simulink model "Working_model_LastVersion24_June_"  (R2020a)
settings: Solver=VariableStepAuto  StartTime=0.0  StopTime=20  RelTol=1e-3
values from neighbouring files (symbols this model uses):
  g = 9.81    [Working_model_LastVersion24_June.m]    (also in model_and_controller.m)
  K = (m_b/(m_b+(Ib/r_b^2)))    (= 0.714285714286)    [Working_model_LastVersion24_June.m]    (also in model_and_controller.m)
  Ts_Outer = 0.1    [Working_model_LastVersion24_June.m]    (also in model_and_controller.m)
undefined symbols (not defined in the file or in its folder): denc_mi, denco12_dis_des, denF, denp_mi, numc_mi, numco12_dis_des, numF, nump_mi
libraries: simulink x1
settings Model: PacingRate=0.500000  Creator=elakz  LastModifiedBy=elakz

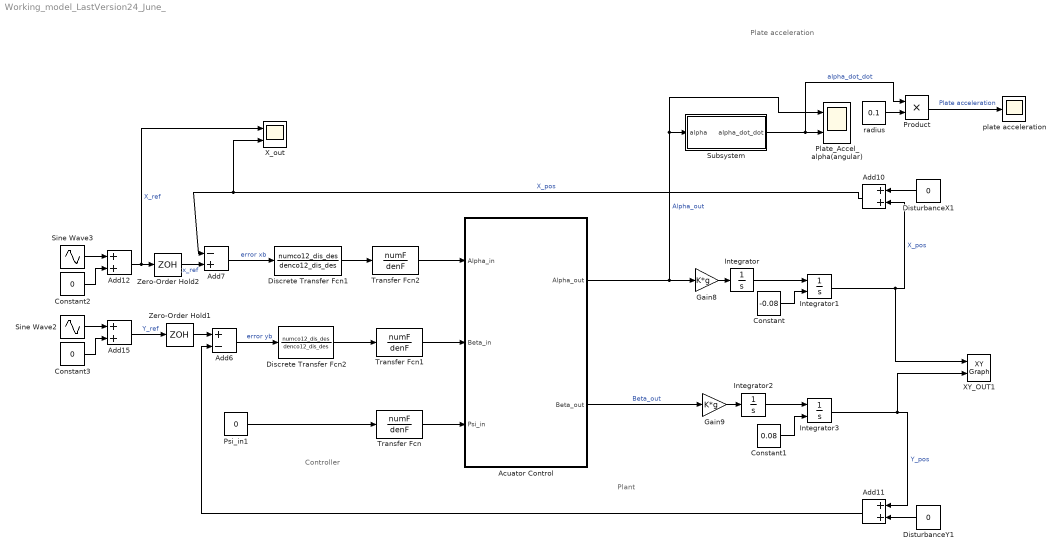
== system Working_model_LastVersion24_June_ ==
  note: Controller
  note: Plant
  note: Plate acceleration
  Acuator Control : Subsystem
  Add{10..12,15} (4 alike) : Sum
  Add6 : Sum  Inputs=+-
  Add7 : Sum  Inputs=-+
  Constant : Constant  Value=-0.08
  Constant1 : Constant  Value=0.08
  Constant2 : Constant  Value=0
  Constant3 : Constant  Value=0
  Discrete Transfer Fcn1 : DiscreteTransferFcn  Numerator=numco12_dis_des  Denominator=denco12_dis_des
  Discrete Transfer Fcn2 : DiscreteTransferFcn  Numerator=numco12_dis_des  Denominator=denco12_dis_des
  DisturbanceX1 : Constant  Value=0
  DisturbanceY1 : Constant  Value=0
  Gain8 : Gain  Gain=K*g
  Gain9 : Gain  Gain=K*g
  Integrator : Integrator
  Integrator1 : Integrator  InitialConditionSource=external  InitialCondition=0.01
  Integrator2 : Integrator
  Integrator3 : Integrator  InitialConditionSource=external  InitialCondition=0.01
  Plate_Accel_alpha(angular) : Scope  NumInputPorts=2
  Product : Product
  Psi_in1 : Constant  Value=0
  Sine Wave2 : Sin  Amplitude=0.1  Frequency=2*pi*0.6  Phase=pi/2  SampleTime=0
  Sine Wave3 : Sin  Amplitude=0.1  Frequency=2*pi*0.6  SampleTime=0
  Subsystem : Subsystem
  Transfer Fcn : TransferFcn  Numerator=numF  Denominator=denF
  Transfer Fcn1 : TransferFcn  Numerator=numF  Denominator=denF
  Transfer Fcn2 : TransferFcn  Numerator=numF  Denominator=denF
  XY_OUT1 : simulink/Sinks/XY Graph  xmin=-0.2  xmax=0.2  ymin=-0.2  ymax=0.2  st=-1
  X_out : Scope  NumInputPorts=2
  Zero-Order Hold1 : ZeroOrderHold  SampleTime=Ts_Outer
  Zero-Order Hold2 : ZeroOrderHold  SampleTime=Ts_Outer
  plate acceleration : Scope
  radius : Constant  Value=0.1
  wires:
  Constant3/1 -> Add15/2
  Constant/1 -> Integrator1/2
  Zero-Order Hold1/1 -> Add6/1
  Integrator3/1 -> XY_OUT1/2, Add11/1  "Y_pos"
  DisturbanceX1/1 -> Add10/1
  Add11/1 -> Add6/2
  Gain8/1 -> Integrator/1
  Add7/1 -> Discrete Transfer Fcn1/1  "error xb"
  Add6/1 -> Discrete Transfer Fcn2/1  "error yb"
  DisturbanceY1/1 -> Add11/2
  Gain9/1 -> Integrator2/1
  Zero-Order Hold2/1 -> Add7/2  "x_ref"
  Integrator1/1 -> XY_OUT1/1, Add10/2  "X_pos"
  Integrator/1 -> Integrator1/1
  Subsystem/1(alpha_dot_dot) -> Product/1, Plate_Accel_alpha(angular)/2  "alpha_dot_dot"
  Constant2/1 -> Add12/2
  Constant1/1 -> Integrator3/2
  Sine Wave3/1 -> Add12/1
  Integrator2/1 -> Integrator3/1
  Add10/1 -> X_out/2, Add7/1  "X_pos"
  Sine Wave2/1 -> Add15/1
  Acuator Control/1(Alpha_out) -> Subsystem/1(alpha), Plate_Accel_alpha(angular)/1, Gain8/1  "Alpha_out"
  Acuator Control/2(Beta_out) -> Gain9/1  "Beta_out"
  Add12/1 -> X_out/1, Zero-Order Hold2/1  "X_ref"
  Transfer Fcn2/1 -> Acuator Control/1(Alpha_in)
  Discrete Transfer Fcn1/1 -> Transfer Fcn2/1
  Transfer Fcn1/1 -> Acuator Control/2(Beta_in)
  Discrete Transfer Fcn2/1 -> Transfer Fcn1/1
  Psi_in1/1 -> Transfer Fcn/1
  Transfer Fcn/1 -> Acuator Control/3(Psi_in)
  radius/1 -> Product/2
  Product/1 -> plate acceleration/1  "Plate acceleration"
  Add15/1 -> Zero-Order Hold1/1  "Y_ref"

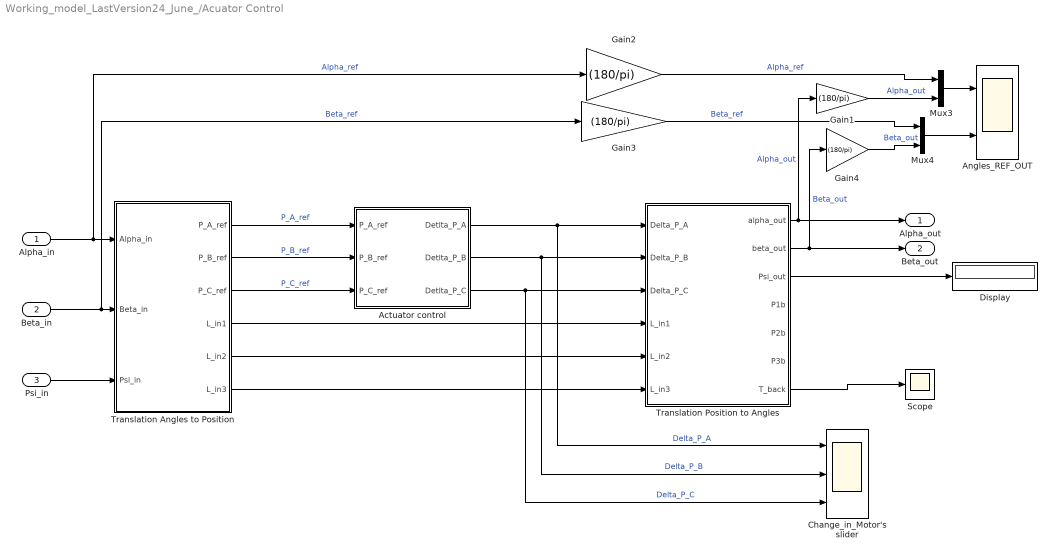
== system Working_model_LastVersion24_June_/Acuator Control ==
  Alpha_in : Inport
  Beta_in : Inport  Port=2
  Psi_in : Inport  Port=3
  Actuator control : Subsystem
  Angles_REF_OUT : Scope  NumInputPorts=2
  Change_in_Motor's slider : Scope  NumInputPorts=3
  Display : Display
  Gain{1..4} (4 alike) : Gain  Gain=(180/pi)
  Mux3 : Mux  Inputs=2
  Mux4 : Mux  Inputs=2
  Scope : Scope
  Translation Angles to Position : Subsystem
  Translation Position to Angles : Subsystem
  Alpha_out : Outport  VectorParamsAs1DForOutWhenUnconnected=off
  Beta_out : Outport  Port=2  VectorParamsAs1DForOutWhenUnconnected=off
  wires:
  Translation Angles to Position/6(L_in3) -> Translation Position to Angles/6(L_in3)
  Translation Angles to Position/1(P_A_ref) -> Actuator control/1(P_A_ref)  "P_A_ref"
  Actuator control/2(Detlta_P_B) -> Change_in_Motor's slider/2, Translation Position to Angles/2(Delta_P_B)  "Delta_P_B"
  Actuator control/3(Detlta_P_C) -> Change_in_Motor's slider/3, Translation Position to Angles/3(Delta_P_C)  "Delta_P_C"
  Translation Angles to Position/2(P_B_ref) -> Actuator control/2(P_B_ref)  "P_B_ref"
  Translation Angles to Position/5(L_in2) -> Translation Position to Angles/5(L_in2)
  Translation Angles to Position/3(P_C_ref) -> Actuator control/3(P_C_ref)  "P_C_ref"
  Translation Angles to Position/4(L_in1) -> Translation Position to Angles/4(L_in1)
  Actuator control/1(Detlta_P_A) -> Change_in_Motor's slider/1, Translation Position to Angles/1(Delta_P_A)  "Delta_P_A"
  Beta_in/1 -> Gain3/1, Translation Angles to Position/2(Beta_in)  "Beta_ref"
  Psi_in/1 -> Translation Angles to Position/3(Psi_in)
  Translation Position to Angles/2(beta_out) -> Gain4/1, Beta_out/1  "Beta_out"
  Translation Position to Angles/1(alpha_out) -> Gain1/1, Alpha_out/1  "Alpha_out"
  Alpha_in/1 -> Gain2/1, Translation Angles to Position/1(Alpha_in)  "Alpha_ref"
  Translation Position to Angles/3(Psi_out) -> Display/1
  Mux3/1 -> Angles_REF_OUT/1
  Mux4/1 -> Angles_REF_OUT/2
  Gain2/1 -> Mux3/1  "Alpha_ref"
  Gain1/1 -> Mux3/2  "Alpha_out"
  Gain3/1 -> Mux4/1  "Beta_ref"
  Gain4/1 -> Mux4/2  "Beta_out"
  Translation Position to Angles/7(T_back) -> Scope/1

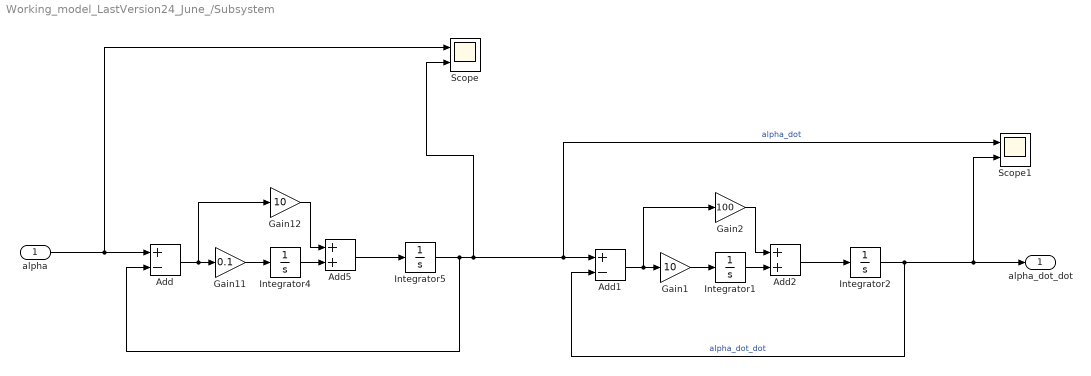
== system Working_model_LastVersion24_June_/Subsystem ==
  alpha : Inport
  Add : Sum  Inputs=+-
  Add1 : Sum  Inputs=+-
  Add2 : Sum
  Add5 : Sum
  Gain1 : Gain  Gain=10
  Gain11 : Gain  Gain=0.1
  Gain12 : Gain  Gain=10
  Gain2 : Gain  Gain=100
  Integrator{1..2,4..5} (4 alike) : Integrator
  Scope : Scope  NumInputPorts=2
  Scope1 : Scope  NumInputPorts=2
  alpha_dot_dot : Outport
  wires:
  Gain11/1 -> Integrator4/1
  Add5/1 -> Integrator5/1
  Gain1/1 -> Integrator1/1
  Integrator4/1 -> Add5/2
  Add/1 -> Gain12/1, Gain11/1
  Gain12/1 -> Add5/1
  Integrator2/1 -> alpha_dot_dot/1, Scope1/2, Add1/2  "alpha_dot_dot"
  Integrator5/1 -> Add/2, Scope/2, Scope1/1, Add1/1  "alpha_dot"
  Integrator1/1 -> Add2/2
  Add1/1 -> Gain2/1, Gain1/1
  Add2/1 -> Integrator2/1
  Gain2/1 -> Add2/1
  alpha/1 -> Scope/1, Add/1

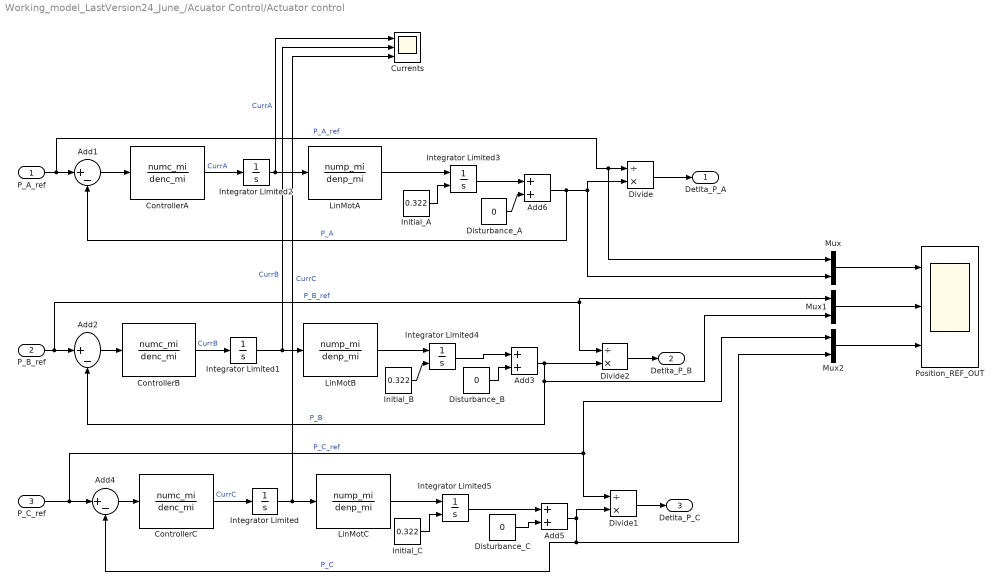
== system Working_model_LastVersion24_June_/Acuator Control/Actuator control ==
  P_A_ref : Inport
  P_B_ref : Inport  Port=2
  P_C_ref : Inport  Port=3
  Add1 : Sum  Inputs=|+-
  Add2 : Sum  Inputs=|+-
  Add3 : Sum
  Add4 : Sum  Inputs=|+-
  Add5 : Sum
  Add6 : Sum
  ControllerA : TransferFcn  Numerator=numc_mi  Denominator=denc_mi
  ControllerB : TransferFcn  Numerator=numc_mi  Denominator=denc_mi
  ControllerC : TransferFcn  Numerator=numc_mi  Denominator=denc_mi
  Currents : Scope  NumInputPorts=3
  Disturbance_A : Constant  Value=0
  Disturbance_B : Constant  Value=0
  Disturbance_C : Constant  Value=0
  Divide : Product  Inputs=/*
  Divide1 : Product  Inputs=/*
  Divide2 : Product  Inputs=/*
  Initial_A : Constant  Value=0.322
  Initial_B : Constant  Value=0.322
  Initial_C : Constant  Value=0.322
  Integrator Limited : Integrator  UpperSaturationLimit=3  LowerSaturationLimit=-3
  Integrator Limited1 : Integrator  UpperSaturationLimit=3  LowerSaturationLimit=-3
  Integrator Limited2 : Integrator  UpperSaturationLimit=3  LowerSaturationLimit=-3
  Integrator Limited3 : Integrator  InitialConditionSource=external  UpperSaturationLimit=1  LowerSaturationLimit=0
  Integrator Limited4 : Integrator  InitialConditionSource=external  UpperSaturationLimit=1  LowerSaturationLimit=0
  Integrator Limited5 : Integrator  InitialConditionSource=external  UpperSaturationLimit=1  LowerSaturationLimit=0
  LinMotA : TransferFcn  Numerator=nump_mi  Denominator=denp_mi
  LinMotB : TransferFcn  Numerator=nump_mi  Denominator=denp_mi
  LinMotC : TransferFcn  Numerator=nump_mi  Denominator=denp_mi
  Mux : Mux  Inputs=2
  Mux1 : Mux  Inputs=2
  Mux2 : Mux  Inputs=2
  Position_REF_OUT : Scope  NumInputPorts=3
  Detlta_P_A : Outport  VectorParamsAs1DForOutWhenUnconnected=off
  Detlta_P_B : Outport  Port=2  VectorParamsAs1DForOutWhenUnconnected=off
  Detlta_P_C : Outport  Port=3  VectorParamsAs1DForOutWhenUnconnected=off
  wires:
  Add6/1 -> Divide/2, Mux/2, Add1/2  "P_A"
  Disturbance_A/1 -> Add6/2
  Add1/1 -> ControllerA/1
  Add2/1 -> ControllerB/1
  Disturbance_B/1 -> Add3/2
  Add3/1 -> Add2/2, Mux1/2, Divide2/2  "P_B"
  Add4/1 -> ControllerC/1
  Disturbance_C/1 -> Add5/2
  Add5/1 -> Divide1/2, Add4/2, Mux2/2  "P_C"
  P_B_ref/1 -> Add2/1, Divide2/1, Mux1/1  "P_B_ref"
  P_A_ref/1 -> Add1/1, Mux/1, Divide/1  "P_A_ref"
  P_C_ref/1 -> Add4/1, Divide1/1, Mux2/1  "P_C_ref"
  Integrator Limited/1 -> Currents/3, LinMotC/1  "CurrC"
  ControllerC/1 -> Integrator Limited/1  "CurrC"
  Integrator Limited1/1 -> LinMotB/1, Currents/2  "CurrB"
  ControllerB/1 -> Integrator Limited1/1  "CurrB"
  Integrator Limited2/1 -> LinMotA/1, Currents/1  "CurrA"
  ControllerA/1 -> Integrator Limited2/1  "CurrA"
  Divide2/1 -> Detlta_P_B/1
  Divide1/1 -> Detlta_P_C/1
  Divide/1 -> Detlta_P_A/1
  Mux1/1 -> Position_REF_OUT/2
  Mux/1 -> Position_REF_OUT/1
  Mux2/1 -> Position_REF_OUT/3
  LinMotA/1 -> Integrator Limited3/1
  Integrator Limited3/1 -> Add6/1
  Initial_A/1 -> Integrator Limited3/2
  Initial_B/1 -> Integrator Limited4/2
  LinMotB/1 -> Integrator Limited4/1
  Integrator Limited4/1 -> Add3/1
  LinMotC/1 -> Integrator Limited5/1
  Initial_C/1 -> Integrator Limited5/2
  Integrator Limited5/1 -> Add5/1

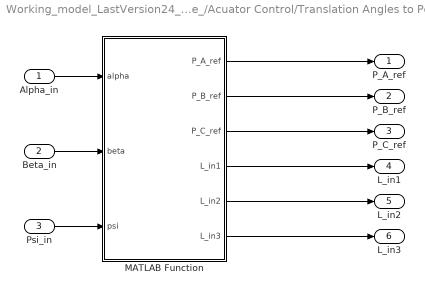
== system Working_model_LastVersion24_June_/Acuator Control/Translation Angles to Position ==
  Alpha_in : Inport
  Beta_in : Inport  Port=2
  Psi_in : Inport  Port=3
  MATLAB Function : MATLAB Function  TreatAsAtomicUnit=on
  P_A_ref : Outport  VectorParamsAs1DForOutWhenUnconnected=off
  P_B_ref : Outport  Port=2  VectorParamsAs1DForOutWhenUnconnected=off
  P_C_ref : Outport  Port=3  VectorParamsAs1DForOutWhenUnconnected=off
  L_in1 : Outport  Port=4  VectorParamsAs1DForOutWhenUnconnected=off
  L_in2 : Outport  Port=5  VectorParamsAs1DForOutWhenUnconnected=off
  L_in3 : Outport  Port=6  VectorParamsAs1DForOutWhenUnconnected=off
  wires:
  Alpha_in/1 -> MATLAB Function/1(alpha)
  MATLAB Function/6(L_in3) -> L_in3/1
  Psi_in/1 -> MATLAB Function/3(psi)
  MATLAB Function/5(L_in2) -> L_in2/1
  MATLAB Function/3(P_C_ref) -> P_C_ref/1
  MATLAB Function/2(P_B_ref) -> P_B_ref/1
  Beta_in/1 -> MATLAB Function/2(beta)
  MATLAB Function/4(L_in1) -> L_in1/1
  MATLAB Function/1(P_A_ref) -> P_A_ref/1

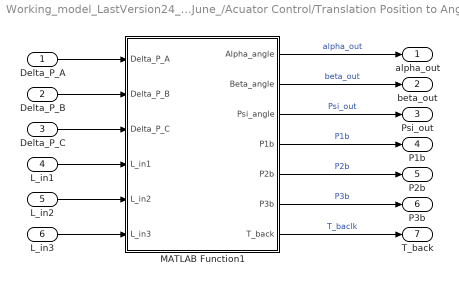
== system Working_model_LastVersion24_June_/Acuator Control/Translation Position to Angles ==
  Delta_P_A : Inport
  Delta_P_B : Inport  Port=2
  Delta_P_C : Inport  Port=3
  L_in1 : Inport  Port=4
  L_in2 : Inport  Port=5
  L_in3 : Inport  Port=6
  MATLAB Function1 : MATLAB Function  TreatAsAtomicUnit=on
  alpha_out : Outport  VectorParamsAs1DForOutWhenUnconnected=off
  beta_out : Outport  Port=2  VectorParamsAs1DForOutWhenUnconnected=off
  Psi_out : Outport  Port=3  VectorParamsAs1DForOutWhenUnconnected=off
  P1b : Outport  Port=4  VectorParamsAs1DForOutWhenUnconnected=off
  P2b : Outport  Port=5  VectorParamsAs1DForOutWhenUnconnected=off
  P3b : Outport  Port=6  VectorParamsAs1DForOutWhenUnconnected=off
  T_back : Outport  Port=7  VectorParamsAs1DForOutWhenUnconnected=off
  wires:
  MATLAB Function1/7(T_back) -> T_back/1  "T_baclk"
  MATLAB Function1/4(P1b) -> P1b/1  "P1b"
  MATLAB Function1/5(P2b) -> P2b/1  "P2b"
  Delta_P_C/1 -> MATLAB Function1/3(Delta_P_C)
  MATLAB Function1/6(P3b) -> P3b/1  "P3b"
  Delta_P_A/1 -> MATLAB Function1/1(Delta_P_A)
  Delta_P_B/1 -> MATLAB Function1/2(Delta_P_B)
  MATLAB Function1/3(Psi_angle) -> Psi_out/1  "Psi_out"
  MATLAB Function1/1(Alpha_angle) -> alpha_out/1  "alpha_out"
  MATLAB Function1/2(Beta_angle) -> beta_out/1  "beta_out"
  L_in3/1 -> MATLAB Function1/6(L_in3)
  L_in1/1 -> MATLAB Function1/4(L_in1)
  L_in2/1 -> MATLAB Function1/5(L_in2)

== matlab function Working_model_LastVersion24_June_/Acuator Control/Translation Angles to Position/MATLAB Function ==
  data: alpha input; beta input; psi input; P_A_ref output; P_B_ref output; P_C_ref output; L_in1 output; L_in2 output; L_in3 output
function [P_A_ref,P_B_ref,P_C_ref,L_in1,L_in2,L_in3] = myfunc(alpha,beta,psi)

%% Rotation matrices

%    Z rotation with angle  psi
RotZ  = [cos(psi) -sin(psi) 0;
         sin(psi)  cos(psi) 0;
          0          0      1]
      
%    Y rotation with angle beta+
RotY  = [cos(beta)       0         sin(beta);
             0           1             0    ;
         -sin(beta)      0        cos(beta)]
    
%    X rotation with angle alpha
RotX  = [1            0                 0    ;
         0        cos(alpha)      -sin(alpha);
         0        sin(alpha)       cos(alpha)]
Rot_BtoP = RotZ*RotY*RotX

%% Specification of the base plate and plate

%Location of motors on the base plate 
r_base = 0.17;               %radii of the base plate (m)
B1     = [r_base; 0; 0]      %position of motor wrt base plate origin
B2     = [-0.5*r_base; (sqrt(3)/2)*r_base; 0]  %120degrees wrt the position of first motor and base plate origin
B3     = [-0.5*r_base; -(sqrt(3)/2)*r_base; 0] %240 degrees wrt first motor and base plate origin

%Location of joints on the plate 
r_plate = 0.17;               %radii of the plate (m)
P1     = [r_plate; 0; 0]      %position of motor wrt base plate origin
P2     = [-0.5*r_plate; (sqrt(3)/2)*r_plate; 0]  %120degrees wrt the position of first motor and base plate origin
P3     = [-0.5*r_plate; -(sqrt(3)/2)*r_plate; 0] %240 degrees wrt first motor and base plate origin

% distance from base plate origin(OXYZ) to plate origin(oxyz)
T = [0; 0; 0.322]                     %30 cm height from (OXYZ) to (oxyz)

%% 
L_in1 = T + (Rot_BtoP*P1)-B1       %change of position of lin motor 1
P_A_ref = sqrt(L_in1(1,1)^2+L_in1(2,1)^2+L_in1(3,1)^2)   %length of L_in1 for passing to motor tf

L_in2 = T + (Rot_BtoP*P2)-B2
P_B_ref = sqrt(L_in2(1,1)^2+L_in2(2,1)^2+L_in2(3,1)^2)

L_in3 = T + (Rot_BtoP*P3)-B3 
P_C_ref = sqrt(L_in3(1,1)^2+L_in3(2,1)^2+L_in3(3,1)^2)
end

== matlab function Working_model_LastVersion24_June_/Acuator Control/Translation Position to Angles/MATLAB Function1 ==
  data: Delta_P_A input; Alpha_angle output; Delta_P_B input; Delta_P_C input; L_in1 input; L_in2 input; L_in3 input; Beta_angle output; Psi_angle output; P1b output; P2b output; P3b output; T_back output
function [Alpha_angle,Beta_angle,Psi_angle,P1b,P2b,P3b,T_back]      = myfunc(Delta_P_A,Delta_P_B,Delta_P_C,L_in1,L_in2,L_in3)



%% Specification of the base plate and plate

%Location of motors on the base plate 
r_base = 0.17;               %radii of the base plate (m)
B1     = [r_base; 0; 0]      %position of motor wrt base plate origin
B2     = [-0.5*r_base; (sqrt(3)/2)*r_base; 0]  %120degrees wrt the position of first motor and base plate origin
B3     = [-0.5*r_base; -(sqrt(3)/2)*r_base; 0] %240 degrees wrt first motor and base plate origin

%Location of joints on the plate 
r_plate = 0.17;               %radii of the plate (m)
P1     = [r_plate; 0; 0];      %position of motor wrt base plate origin
P2     = [-0.5*r_plate; (sqrt(3)/2)*r_plate; 0];  %120degrees wrt the position of first motor and base plate origin
P3     = [-0.5*r_plate; -(sqrt(3)/2)*r_plate; 0]; %240 degrees wrt first motor and base plate origin

% distance from base plate origin(OXYZ) to plate origin(oxyz)
T = [0; 0; 0.322]                     %30 cm height from (OXYZ) to (oxyz)

%actuator plate connections in base frame
% P1b= B1+(L_in1)-T;
% P2b= B2+(L_in2)-T;
% P3b= B3+(L_in3)-T;

P1b= B1+(L_in1*(Delta_P_A))-T;
P2b= B2+(L_in2*(Delta_P_B))-T;
P3b= B3+(L_in3*(Delta_P_C))-T;

%base frame unit vectors
UnitX=[1;0;0];
UnitY=[0;1;0];
UnitZ=[0;0;1];
UnitXp=P1b/sqrt(dot(P1b,P1b));
UnitZp=cross(UnitXp,P3b);
UnitZp=UnitZp/sqrt(dot(UnitZp,UnitZp)); %now length 1
UnitYp=cross(UnitXp,UnitZp);

%this is according to https://en.wikipedia.org/wiki/Euler_angles, Tait-Bryn
%angles

Beta_angle=asin(-UnitXp(3))
Psi_angle=asin(UnitXp(2)/sqrt(1-UnitXp(3)^2))
Alpha_angle=asin(UnitYp(3)/sqrt(1-UnitXp(3)^2))

%Calculating rotation matrix with above angles
RotZ1  = [cos(Psi_angle) -sin(Psi_angle) 0;
         sin(Psi_angle)  cos(Psi_angle) 0;
          0          0      1];
      
%    Y rotation with angle beta
RotY1  = [cos(Beta_angle)       0         sin(Beta_angle);
             0                           1             0    ;
         -sin(Beta_angle)      0        cos(Beta_angle)];
    
%    X rotation with angle alpha
RotX1  = [1            0                                 0    ;
         0        cos(Alpha_angle)      -sin(Alpha_angle);
         0        sin(Alpha_angle)       cos(Alpha_angle)];

% Calculating back the T matrix which was the height between the base plate
% and plate. They must be the same.
Rm_times_P = RotZ1*RotY1*RotX1
T_back = L_in1+B1-(Rm_times_P*P1)

end
